simulink model "Clark_Park_Transform"  (R2025a)
settings: Solver=FixedStepDiscrete  StartTime=0.0  StopTime=0.1  FixedStep=1e-06  RelTol=1e-3
libraries: simulink x1
settings Model: Creator=jicai  LastModifiedBy=jicai

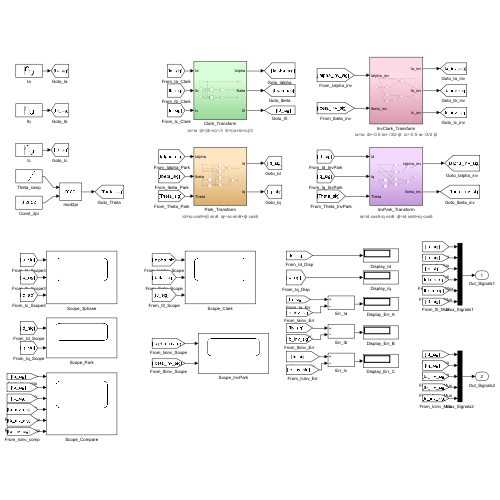
[thumbnail: Simulink's stored preview of the top-level diagram]
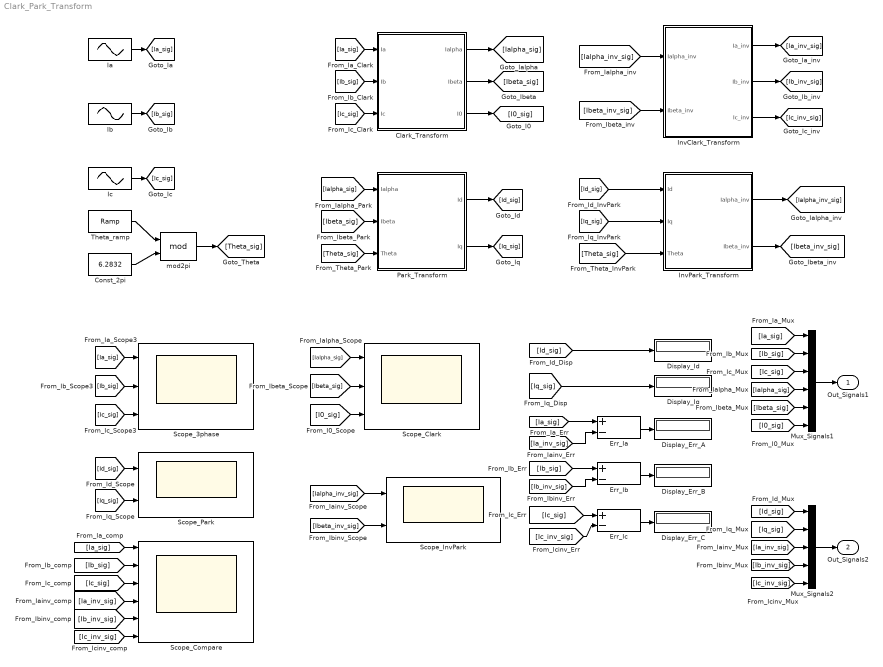
== system Clark_Park_Transform ==
  Clark_Transform : Subsystem
      settings: AttributesFormatString="iα=ia  iβ=(ib-ic)/√3  i0=(ia+ib+ic)/3"
  Const_2pi : Constant  Value=6.2832
  Display_Err_A : Display
  Display_Err_B : Display
  Display_Err_C : Display
  Display_Id : Display
  Display_Iq : Display
  Err_Ia : Sum  Inputs=+-
  Err_Ib : Sum  Inputs=+-
  Err_Ic : Sum  Inputs=+-
  Ia : Sin  Amplitude=10  Frequency=314.1593  Phase=1.5708  SampleTime=1e-06
  Ib : Sin  Amplitude=10  Frequency=314.1593  Phase=-0.5236  SampleTime=1e-06
  Ic : Sin  Amplitude=10  Frequency=314.1593  Phase=3.6652  SampleTime=1e-06
  InvClark_Transform : Subsystem
      settings: AttributesFormatString="ia=iα  ib=-0.5·iα+√3/2·iβ  ic=-0.5·iα-√3/2·iβ"
  InvPark_Transform : Subsystem
      settings: AttributesFormatString="iα=id·cosθ-iq·sinθ  iβ=id·sinθ+iq·cosθ"
  Mux_Signals1 : Mux  Inputs=6
  Mux_Signals2 : Mux  Inputs=5
  Park_Transform : Subsystem
      settings: AttributesFormatString="id=iα·cosθ+iβ·sinθ  iq=-iα·sinθ+iβ·cosθ"
  Scope_3phase : Scope  NumInputPorts=3
      settings: ActiveDisplayYMinimum=-12.49999999990569  ActiveDisplayYMaximum=12.499999999914563
  Scope_Clark : Scope  NumInputPorts=3
      settings: ActiveDisplayYMinimum=-12.49999999990569  ActiveDisplayYMaximum=12.499999999914563
  Scope_Compare : Scope  NumInputPorts=6
      settings: ActiveDisplayYMinimum=-0.13438836994152226  ActiveDisplayYMaximum=6.6492064772059258
  Scope_InvPark : Scope  NumInputPorts=2
  Scope_Park : Scope  NumInputPorts=2
      settings: ActiveDisplayYMinimum=-1.24997458200582  ActiveDisplayYMaximum=11.24999717571338
  Theta_ramp : simulink/Sources/Ramp  slope=314.1593  start=0  InitialOutput=0
  mod2pi : Math  Operator=mod
  Out_Signals1 : Outport
  Out_Signals2 : Outport  Port=2
  wires:
  Ia/1 -> [Ia_sig]
  Ib/1 -> [Ib_sig]
  Ic/1 -> [Ic_sig]
  Const_2pi/1 -> mod2pi/2
  Theta_ramp/1 -> mod2pi/1
  mod2pi/1 -> [Theta_sig]
  [Ia_sig] -> Clark_Transform/1(Ia)
  [Ib_sig] -> Clark_Transform/2(Ib)
  [Ic_sig] -> Clark_Transform/3(Ic)
  Clark_Transform/1(Ialpha) -> [Ialpha_sig]
  Clark_Transform/2(Ibeta) -> [Ibeta_sig]
  Clark_Transform/3(I0) -> [I0_sig]
  [Ialpha_sig] -> Park_Transform/1(Ialpha)
  [Ibeta_sig] -> Park_Transform/2(Ibeta)
  [Theta_sig] -> Park_Transform/3(Theta)
  Park_Transform/1(Id) -> [Id_sig]
  Park_Transform/2(Iq) -> [Iq_sig]
  [Id_sig] -> InvPark_Transform/1(Id)
  [Iq_sig] -> InvPark_Transform/2(Iq)
  [Theta_sig] -> InvPark_Transform/3(Theta)
  InvPark_Transform/1(Ialpha_inv) -> [Ialpha_inv_sig]
  InvPark_Transform/2(Ibeta_inv) -> [Ibeta_inv_sig]
  [Ialpha_inv_sig] -> InvClark_Transform/1(Ialpha_inv)
  [Ibeta_inv_sig] -> InvClark_Transform/2(Ibeta_inv)
  InvClark_Transform/1(Ia_inv) -> [Ia_inv_sig]
  InvClark_Transform/2(Ib_inv) -> [Ib_inv_sig]
  InvClark_Transform/3(Ic_inv) -> [Ic_inv_sig]
  [Ia_sig] -> Scope_3phase/1
  [Ib_sig] -> Scope_3phase/2
  [Ic_sig] -> Scope_3phase/3
  [Ialpha_sig] -> Scope_Clark/1
  [Ibeta_sig] -> Scope_Clark/2
  [I0_sig] -> Scope_Clark/3
  [Id_sig] -> Scope_Park/1
  [Iq_sig] -> Scope_Park/2
  [Ialpha_inv_sig] -> Scope_InvPark/1
  [Ibeta_inv_sig] -> Scope_InvPark/2
  [Ia_sig] -> Scope_Compare/1
  [Ib_sig] -> Scope_Compare/2
  [Ic_sig] -> Scope_Compare/3
  [Ia_inv_sig] -> Scope_Compare/4
  [Ib_inv_sig] -> Scope_Compare/5
  [Ic_inv_sig] -> Scope_Compare/6
  [Id_sig] -> Display_Id/1
  [Iq_sig] -> Display_Iq/1
  [Ia_sig] -> Err_Ia/1
  [Ia_inv_sig] -> Err_Ia/2
  [Ib_sig] -> Err_Ib/1
  [Ib_inv_sig] -> Err_Ib/2
  [Ic_sig] -> Err_Ic/1
  [Ic_inv_sig] -> Err_Ic/2
  Err_Ia/1 -> Display_Err_A/1
  Err_Ib/1 -> Display_Err_B/1
  Err_Ic/1 -> Display_Err_C/1
  [Ia_sig] -> Mux_Signals1/1
  [Ib_sig] -> Mux_Signals1/2
  [Ic_sig] -> Mux_Signals1/3
  [Ialpha_sig] -> Mux_Signals1/4
  [Ibeta_sig] -> Mux_Signals1/5
  [I0_sig] -> Mux_Signals1/6
  Mux_Signals1/1 -> Out_Signals1/1
  [Id_sig] -> Mux_Signals2/1
  [Iq_sig] -> Mux_Signals2/2
  [Ia_inv_sig] -> Mux_Signals2/3
  [Ib_inv_sig] -> Mux_Signals2/4
  [Ic_inv_sig] -> Mux_Signals2/5
  Mux_Signals2/1 -> Out_Signals2/1

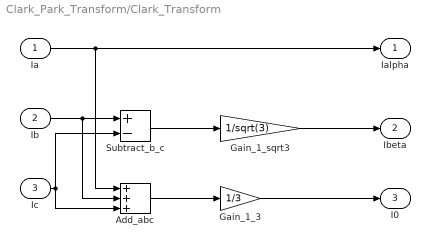
== system Clark_Park_Transform/Clark_Transform ==
  Ia : Inport
  Ib : Inport  Port=2
  Ic : Inport  Port=3
  Add_abc : Sum  Inputs=+++
  Gain_1_3 : Gain  Gain=1/3
  Gain_1_sqrt3 : Gain  Gain=1/sqrt(3)
  Subtract_b_c : Sum  Inputs=+-
  Ialpha : Outport
  Ibeta : Outport  Port=2
  I0 : Outport  Port=3
  wires:
  Ia/1 -> Ialpha/1, Add_abc/1
  Ib/1 -> Subtract_b_c/1, Add_abc/2
  Ic/1 -> Subtract_b_c/2, Add_abc/3
  Subtract_b_c/1 -> Gain_1_sqrt3/1
  Gain_1_sqrt3/1 -> Ibeta/1
  Add_abc/1 -> Gain_1_3/1
  Gain_1_3/1 -> I0/1

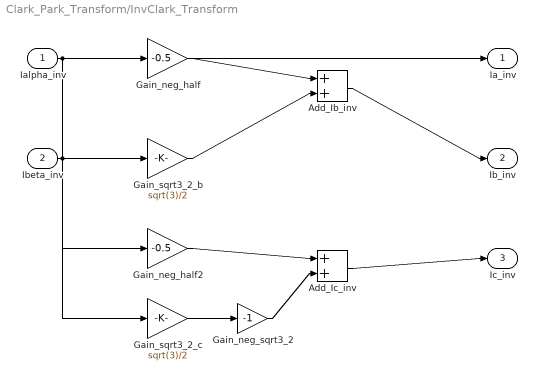
== system Clark_Park_Transform/InvClark_Transform ==
  Ialpha_inv : Inport
  Ibeta_inv : Inport  Port=2
  Add_Ib_inv : Sum
  Add_Ic_inv : Sum
  Gain_neg_half : Gain  Gain=-0.5
  Gain_neg_half2 : Gain  Gain=-0.5
  Gain_neg_sqrt3_2 : Gain  Gain=-1
  Gain_sqrt3_2_b : Gain  Gain=sqrt(3)/2
  Gain_sqrt3_2_c : Gain  Gain=sqrt(3)/2
  Ia_inv : Outport
  Ib_inv : Outport  Port=2
  Ic_inv : Outport  Port=3
  wires:
  Ialpha_inv/1 -> Ia_inv/1, Gain_neg_half/1, Gain_neg_half2/1
  Ibeta_inv/1 -> Gain_sqrt3_2_b/1, Gain_sqrt3_2_c/1
  Gain_neg_half/1 -> Add_Ib_inv/1
  Gain_sqrt3_2_b/1 -> Add_Ib_inv/2
  Add_Ib_inv/1 -> Ib_inv/1
  Gain_sqrt3_2_c/1 -> Gain_neg_sqrt3_2/1
  Gain_neg_half2/1 -> Add_Ic_inv/1
  Gain_neg_sqrt3_2/1 -> Add_Ic_inv/2
  Add_Ic_inv/1 -> Ic_inv/1

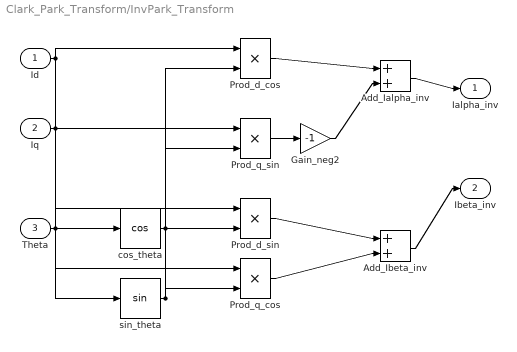
== system Clark_Park_Transform/InvPark_Transform ==
  Id : Inport
  Iq : Inport  Port=2
  Theta : Inport  Port=3
  Add_Ialpha_inv : Sum
  Add_Ibeta_inv : Sum
  Gain_neg2 : Gain  Gain=-1
  Prod_d_cos : Product  Inputs=**
  Prod_d_sin : Product  Inputs=**
  Prod_q_cos : Product  Inputs=**
  Prod_q_sin : Product  Inputs=**
  cos_theta : Trigonometry  Operator=cos
  sin_theta : Trigonometry
  Ialpha_inv : Outport
  Ibeta_inv : Outport  Port=2
  wires:
  Theta/1 -> cos_theta/1, sin_theta/1
  Id/1 -> Prod_d_cos/1, Prod_d_sin/1
  cos_theta/1 -> Prod_d_cos/2, Prod_q_cos/2
  Iq/1 -> Prod_q_sin/1, Prod_q_cos/1
  sin_theta/1 -> Prod_q_sin/2, Prod_d_sin/2
  Prod_q_sin/1 -> Gain_neg2/1
  Gain_neg2/1 -> Add_Ialpha_inv/2
  Prod_d_cos/1 -> Add_Ialpha_inv/1
  Add_Ialpha_inv/1 -> Ialpha_inv/1
  Prod_d_sin/1 -> Add_Ibeta_inv/1
  Prod_q_cos/1 -> Add_Ibeta_inv/2
  Add_Ibeta_inv/1 -> Ibeta_inv/1

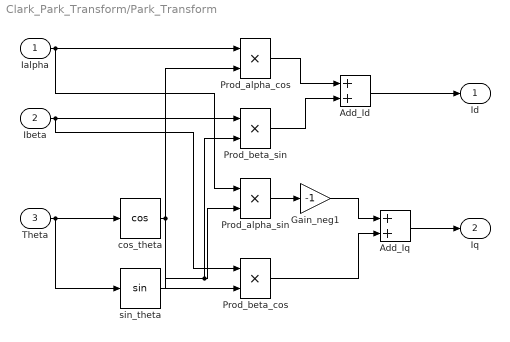
== system Clark_Park_Transform/Park_Transform ==
  Ialpha : Inport
  Ibeta : Inport  Port=2
  Theta : Inport  Port=3
  Add_Id : Sum
  Add_Iq : Sum
  Gain_neg1 : Gain  Gain=-1
  Prod_alpha_cos : Product  Inputs=**
  Prod_alpha_sin : Product  Inputs=**
  Prod_beta_cos : Product  Inputs=**
  Prod_beta_sin : Product  Inputs=**
  cos_theta : Trigonometry  Operator=cos
  sin_theta : Trigonometry
  Id : Outport
  Iq : Outport  Port=2
  wires:
  Theta/1 -> cos_theta/1, sin_theta/1
  Ialpha/1 -> Prod_alpha_cos/1, Prod_alpha_sin/1
  cos_theta/1 -> Prod_alpha_cos/2, Prod_beta_cos/2
  Ibeta/1 -> Prod_beta_sin/1, Prod_beta_cos/1
  sin_theta/1 -> Prod_beta_sin/2, Prod_alpha_sin/2
  Prod_alpha_cos/1 -> Add_Id/1
  Prod_beta_sin/1 -> Add_Id/2
  Add_Id/1 -> Id/1
  Prod_alpha_sin/1 -> Gain_neg1/1
  Gain_neg1/1 -> Add_Iq/1
  Prod_beta_cos/1 -> Add_Iq/2
  Add_Iq/1 -> Iq/1
